simulink model "MPCARX"  (R2019a)
settings: Solver=VariableStepAuto  StartTime=0.0  StopTime=10.0  RelTol=1e-3
InitFcn:
  | run('prepareSim.m')
libraries: delay x2
settings Model: Creator=wangz  LastModifiedBy=wangz

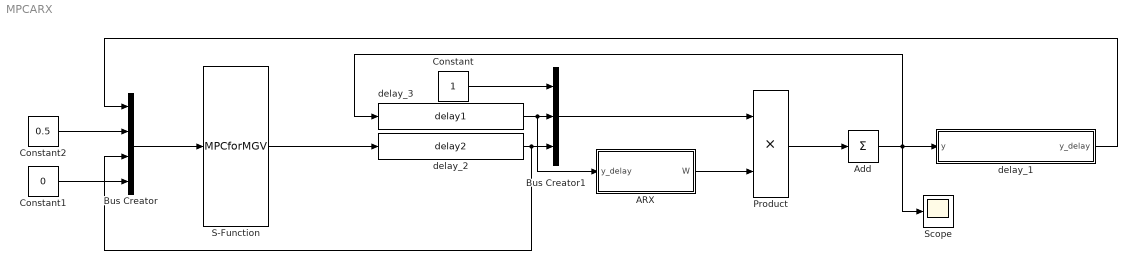
== system MPCARX ==
  ARX : MATLAB Function  TreatAsAtomicUnit=on
  Add : Sum  Inputs=+
  Bus Creator : BusCreator  Inputs=4
  Bus Creator1 : BusCreator  Inputs=3
  Constant : Constant
  Constant1 : Constant  Value=0
  Constant2 : Constant  Value=0.5
  Product : Product
  S-Function : S-Function  FunctionName=MPCforMGV  SFunctionDeploymentMode=off  EnableBusSupport=off
  Scope : Scope
  delay_1 : Subsystem
  delay_2 : delay/delay2  SystemSampleTime=-1
  "delay_3 " : delay/delay1   SystemSampleTime=-1
  wires:
  ARX/1(W) -> Product/2
  Product/1 -> Add/1
  Bus Creator1/1 -> Product/1
  "delay_3 "/1 -> ARX/1(y_delay), Bus Creator1/2
  Constant/1 -> Bus Creator1/1
  delay_2/1 -> Bus Creator/3, Bus Creator1/3
  S-Function/1 -> delay_2/1
  Add/1 -> Scope/1, delay_1/1("y "), "delay_3 "/1
  Bus Creator/1 -> S-Function/1
  delay_1/1(y_delay) -> Bus Creator/1
  Constant1/1 -> Bus Creator/4
  Constant2/1 -> Bus Creator/2

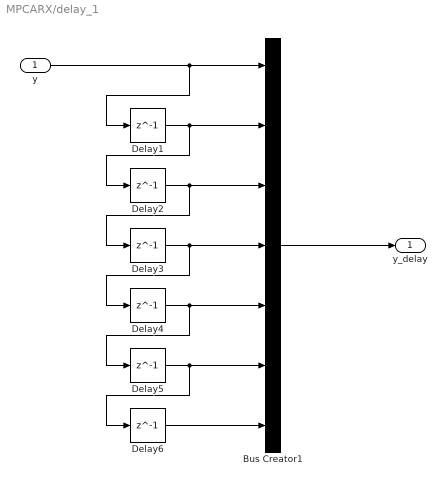
== system MPCARX/delay_1 ==
  "y " : Inport
  Bus Creator1 : BusCreator  Inputs=7
  Delay{1..6} (6 alike) : Delay  DelayLength=1
  y_delay : Outport
  wires:
  "y "/1 -> Bus Creator1/1, Delay1/1
  Delay2/1 -> Bus Creator1/3, Delay3/1
  Delay5/1 -> Bus Creator1/6, Delay6/1
  Delay6/1 -> Bus Creator1/7
  Delay3/1 -> Bus Creator1/4, Delay4/1
  Delay4/1 -> Delay5/1, Bus Creator1/5
  Bus Creator1/1 -> y_delay/1
  Delay1/1 -> Delay2/1, Bus Creator1/2

== matlab function MPCARX/ARX ==
  settings: updateMethod=DISCRETE
  data: W output; y_delay input; model parameter
function W = fcn(y_delay, model)

Wtemp=ARXModel([y_delay(1),y_delay(2)],model);
W=[Wtemp(1) Wtemp(2) Wtemp(3) Wtemp(4) Wtemp(5) Wtemp(6) Wtemp(7) Wtemp(8) Wtemp(9) Wtemp(10) Wtemp(11)]';
